simulink model "blocosnaolinear"  (R2023b)
settings: Solver=VariableStepAuto  StartTime=0.0  StopTime=10.0  RelTol=1e-3
values from neighbouring files (symbols this model uses):
  k1 = 6.01    [q9.m]
  k2 = 0.8433    [q9.m]
  k3 = 0.1123    [q9.m]
undefined symbols (not defined in the file or in its folder): Caf0, FV0
settings Model: Creator=Geovanne  LastModifiedBy=Geovanne

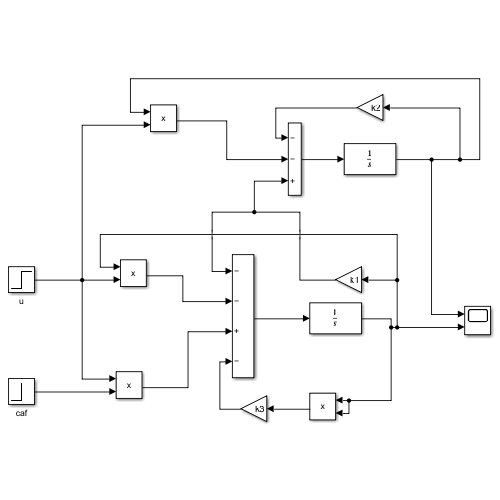
[thumbnail: Simulink's stored preview of the top-level diagram]
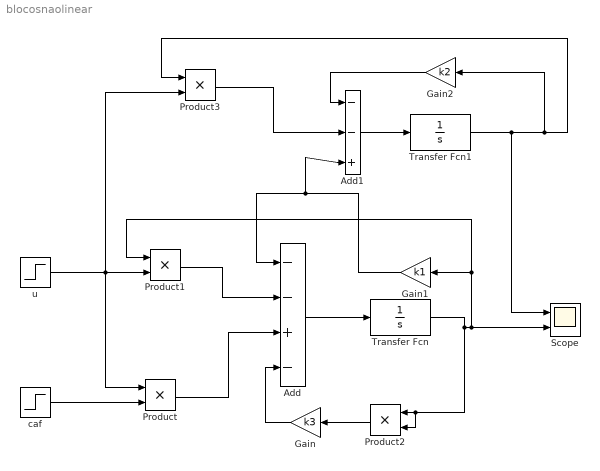
== system blocosnaolinear ==
  Add : Sum  Inputs=--+-
  Add1 : Sum  Inputs=--+
  Gain : Gain  Gain=k3
  Gain1 : Gain  Gain=k1
  Gain2 : Gain  Gain=k2
  Product{,1..3} (4 alike) : Product
  Scope : Scope  NumInputPorts=2
  Transfer Fcn : TransferFcn  Denominator=[1 0]
  Transfer Fcn1 : TransferFcn  Denominator=[1 0]
  caf : Step  Time=0  After=Caf0  SampleTime=0
  u : Step  Time=0  After=FV0  SampleTime=0
  wires:
  caf/1 -> Product/2
  u/1 -> Product3/2, Product1/2, Product/1
  Add/1 -> Transfer Fcn/1
  Transfer Fcn/1 -> Product2/2, Product2/1, Scope/2, Gain1/1, Product1/1
  Product2/1 -> Gain/1
  Gain1/1 -> Add/1, Add1/3
  Gain/1 -> Add/4
  Product1/1 -> Add/2
  Product/1 -> Add/3
  Add1/1 -> Transfer Fcn1/1
  Transfer Fcn1/1 -> Gain2/1, Product3/1, Scope/1
  Gain2/1 -> Add1/1
  Product3/1 -> Add1/2
